simulink model "Project2"  (R2021a)
settings: Solver=VariableStepAuto  StartTime=0.0  StopTime=10.0  RelTol=1e-3
libraries: simulink x1
settings Model: Creator=alan saji  LastModifiedBy=alan saji

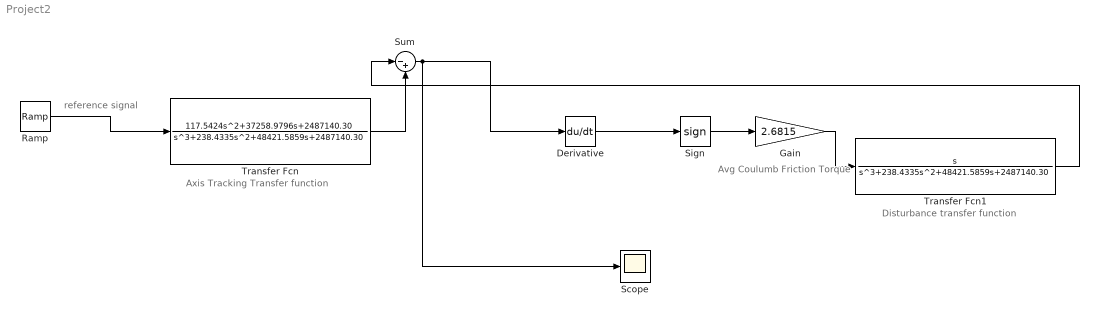
== system Project2 ==
  note: Axis Tracking Transfer function
  note: Disturbance transfer function
  note: Avg Coulumb Friction Torque
  note: reference signal
  Derivative : Derivative
  Gain : Gain  Gain=2.6815
  Ramp : simulink/Sources/Ramp  slope=1  start=0  InitialOutput=0
  Scope : Scope
  Sign : Signum
  Sum : Sum  Inputs=|-+
  Transfer Fcn : TransferFcn  Numerator=[117.5424 37258.9796 2487140.30]  Denominator=[1 238.4335 48421.5859 2487140.30]
  Transfer Fcn1 : TransferFcn  Numerator=[1 0]  Denominator=[1 238.4335 48421.5859 2487140.30]
  wires:
  Sign/1 -> Gain/1
  Derivative/1 -> Sign/1
  Ramp/1 -> Transfer Fcn/1
  Transfer Fcn/1 -> Sum/2
  Sum/1 -> Scope/1, Derivative/1
  Gain/1 -> Transfer Fcn1/1
  Transfer Fcn1/1 -> Sum/1
